simulink library "marine_gnc"  (Simulink 7.4)
settings: Solver=ode45  SolverMode=SingleTasking  StartTime=0.0  StopTime=10.0  RelTol=1e-3
undefined symbols (not defined in the file or in its folder): CN_data, CX_data, CY_data, D, G, K_supply, kt2ms, M, MA, magnitude, marine, Models, MRB, order, pathlength, RAO_Amp, RAO_Dir, RAO_Freq, RAO_Phase, RAO_Vel, RAO_yaw_back, RAO_yaw_quant, RAO_yaw_quantization_flag, rho_a, Semi, sub, T_supply, table, Tanker, vessel, Vessels
libraries: marine_gnc x64, simulink x39, cybersealib x1
(part 4 of 6)

== system marine_gnc/Models/Control Surfaces/Rudder ==
  note: Lift
  note: Drag
  "Alpha_eff " : Inport  OutDataType=sfix(16)  OutScaling=2^0
  Vrel : Inport  Port=2  OutDataType=sfix(16)  OutScaling=2^0
  Constant1 : Constant  Value=CD0  OutDataType=sfix(16)  OutScaling=2^0
  Math Function : Math  Operator=square  OutDataType=sfix(16)  OutScaling=2^0  SaturateOnIntegerOverflow=on
  Mux2 : Mux
  Product1 : Product  Inputs=**  OutDataType=sfix(16)  OutScaling=2^0  SaturateOnIntegerOverflow=on  InputSameDT=on  OutDataTypeStr=Inherit: Same as first input
  Product2 : Product  OutDataType=sfix(16)  OutScaling=2^0  SaturateOnIntegerOverflow=on  InputSameDT=on  OutDataTypeStr=Inherit: Same as first input
  Product4 : Product  OutDataType=sfix(16)  OutScaling=2^0  SaturateOnIntegerOverflow=on  InputSameDT=on  OutDataTypeStr=Inherit: Same as first input
  Saturation : Saturate  UpperLimit=stall  LowerLimit=-stall
  Sum1 : Sum  Inputs=|++  OutDataType=sfix(16)  OutScaling=2^0  SaturateOnIntegerOverflow=on  InputSameDT=on  OutDataTypeStr=Inherit: Same as first input
  "gain " : Gain  Gain=1/(0.9*pi*ar)  ParameterDataType=sfix(16)  ParameterScaling=2^0  OutDataType=sfix(16)  OutScaling=2^0  SaturateOnIntegerOverflow=on  OutDataTypeStr=Inherit: Same as input  ParamDataTypeStr=Inherit: Same as input
  gain 1 : Gain  Gain=dCL  ParameterDataType=sfix(16)  ParameterScaling=2^0  OutDataType=sfix(16)  OutScaling=2^0  SaturateOnIntegerOverflow=on  OutDataTypeStr=Inherit: Same as input  ParamDataTypeStr=Inherit: Same as input
  gain 2 : Gain  Gain=-1  ParameterDataType=sfix(16)  ParameterScaling=2^0  OutDataType=sfix(16)  OutScaling=2^0  SaturateOnIntegerOverflow=on  OutDataTypeStr=Inherit: Same as input  ParamDataTypeStr=Inherit: Same as input
  pi/(2*stall)2 : Gain  Gain=0.5*rho*A  ParameterDataType=sfix(16)  ParameterScaling=2^0  OutDataType=sfix(16)  OutScaling=2^0  SaturateOnIntegerOverflow=on  OutDataTypeStr=Inherit: Same as input  ParamDataTypeStr=Inherit: Same as input
  pi/(2*stall)6 : Gain  Gain=-(VCG-0.5*sp)  ParameterDataType=sfix(16)  ParameterScaling=2^0  OutDataType=sfix(16)  OutScaling=2^0  SaturateOnIntegerOverflow=on  OutDataTypeStr=Inherit: Same as input  ParamDataTypeStr=Inherit: Same as input
  pi/(2*stall)7 : Gain  Gain=-LCG  ParameterDataType=sfix(16)  ParameterScaling=2^0  OutDataType=sfix(16)  OutScaling=2^0  SaturateOnIntegerOverflow=on  OutDataTypeStr=Inherit: Same as input  ParamDataTypeStr=Inherit: Same as input
  "[XYKN]'" : Outport  OutDataType=sfix(16)  OutScaling=2^0
  wires:
  Product1/1 -> pi/(2*stall)2/1
  Vrel/1 -> Product1/2, Product1/1
  Constant1/1 -> Sum1/2
  "gain "/1 -> Sum1/1
  Math Function/1 -> "gain "/1
  Sum1/1 -> Product4/1
  pi/(2*stall)2/1 -> Product2/2, Product4/2
  Product4/1 -> gain 2/1
  gain 2/1 -> Mux2/1
  Mux2/1 -> "[XYKN]'"/1
  pi/(2*stall)6/1 -> Mux2/3
  Product2/1 -> Mux2/2, pi/(2*stall)6/1, pi/(2*stall)7/1
  pi/(2*stall)7/1 -> Mux2/4
  gain 1/1 -> Product2/1, Math Function/1
  Saturation/1 -> gain 1/1
  "Alpha_eff "/1 -> Saturation/1

== system marine_gnc/Models/Control Surfaces/Rudder  forces 4-DOF ==
  Lift : Inport  OutDataType=sfix(16)  OutScaling=2^0
  Drag : Inport  Port=2  OutDataType=sfix(16)  OutScaling=2^0
  Constant : Constant  Value=LCG  OutDataType=sfix(16)  OutScaling=2^0
  Constant2 : Constant  Value=rr  OutDataType=sfix(16)  OutScaling=2^0
  Gain : Gain  Gain=-1  ParameterDataType=sfix(16)  ParameterScaling=2^0  OutDataType=sfix(16)  OutScaling=2^0  SaturateOnIntegerOverflow=on  OutDataTypeStr=Inherit: Same as input  ParamDataTypeStr=Inherit: Same as input
  Gain1 : Gain  Gain=-1  ParameterDataType=sfix(16)  ParameterScaling=2^0  OutDataType=sfix(16)  OutScaling=2^0  SaturateOnIntegerOverflow=on  OutDataTypeStr=Inherit: Same as input  ParamDataTypeStr=Inherit: Same as input
  Product1 : Product  OutDataType=sfix(16)  OutScaling=2^0  SaturateOnIntegerOverflow=on  InputSameDT=on  OutDataTypeStr=Inherit: Same as first input
  Product2 : Product  OutDataType=sfix(16)  OutScaling=2^0  SaturateOnIntegerOverflow=on  InputSameDT=on  OutDataTypeStr=Inherit: Same as first input
  X : Outport  OutDataType=sfix(16)  OutScaling=2^0
  Y : Outport  Port=2  OutDataType=sfix(16)  OutScaling=2^0
  K : Outport  Port=3  OutDataType=sfix(16)  OutScaling=2^0
  N : Outport  Port=4  OutDataType=sfix(16)  OutScaling=2^0
  wires:
  Gain/1 -> X/1
  Drag/1 -> Gain/1
  Gain1/1 -> Product2/1, Product1/1
  Product2/1 -> K/1
  Constant2/1 -> Product2/2
  Lift/1 -> Y/1, Gain1/1
  Constant/1 -> Product1/2
  Product1/1 -> N/1

== system marine_gnc/Models/Control Surfaces/Stabilizer Fins forces 4-DOF ==
  Nf : Inport  OutDataType=sfix(16)  OutScaling=2^0
  Tf : Inport  Port=2  OutDataType=sfix(16)  OutScaling=2^0
  Constant : Constant  Value=FCG  OutDataType=sfix(16)  OutScaling=2^0
  Constant1 : Constant  Value=sinB  OutDataType=sfix(16)  OutScaling=2^0
  Constant2 : Constant  Value=rf  OutDataType=sfix(16)  OutScaling=2^0
  Gain : Gain  Gain=-1  ParameterDataType=sfix(16)  ParameterScaling=2^0  OutDataType=sfix(16)  OutScaling=2^0  SaturateOnIntegerOverflow=on  OutDataTypeStr=Inherit: Same as input  ParamDataTypeStr=Inherit: Same as input
  Gain1 : Gain  Gain=-2  ParameterDataType=sfix(16)  ParameterScaling=2^0  OutDataType=sfix(16)  OutScaling=2^0  SaturateOnIntegerOverflow=on  OutDataTypeStr=Inherit: Same as input  ParamDataTypeStr=Inherit: Same as input
  Product : Product  Inputs=3  OutDataType=sfix(16)  OutScaling=2^0  SaturateOnIntegerOverflow=on  InputSameDT=on  OutDataTypeStr=Inherit: Same as first input
  Product1 : Product  OutDataType=sfix(16)  OutScaling=2^0  SaturateOnIntegerOverflow=on  InputSameDT=on  OutDataTypeStr=Inherit: Same as first input
  Product2 : Product  OutDataType=sfix(16)  OutScaling=2^0  SaturateOnIntegerOverflow=on  InputSameDT=on  OutDataTypeStr=Inherit: Same as first input
  X : Outport  OutDataType=sfix(16)  OutScaling=2^0
  Y : Outport  Port=2  OutDataType=sfix(16)  OutScaling=2^0
  K : Outport  Port=3  OutDataType=sfix(16)  OutScaling=2^0
  N : Outport  Port=4  OutDataType=sfix(16)  OutScaling=2^0
  wires:
  Product1/1 -> Y/1
  Product/1 -> N/1
  Constant/1 -> Product/3
  Constant1/1 -> Product/1, Product1/2
  Nf/1 -> Product/2, Gain1/1, Product1/1
  Constant2/1 -> Product2/2
  Product2/1 -> K/1
  Gain1/1 -> Product2/1
  Tf/1 -> Gain/1
  Gain/1 -> X/1

== system marine_gnc/Models/Control Surfaces/Steady State Hydrofoil ==
  Ang : Inport  OutDataType=sfix(16)  OutScaling=2^0
  "Vf " : Inport  Port=2  OutDataType=sfix(16)  OutScaling=2^0
  Constant1 : Constant  Value=CD0  OutDataType=sfix(16)  OutScaling=2^0
  Gain : Gain  Gain=0.5*rho*A  ParameterDataType=sfix(16)  ParameterScaling=2^0  OutDataType=sfix(16)  OutScaling=2^0  SaturateOnIntegerOverflow=on  OutDataTypeStr=Inherit: Same as input  ParamDataTypeStr=Inherit: Same as input
  Lookup Table CL(Ang) : Lookup  InputValues=AE  Table=CLAE  LookUpMeth=Interpolation-Use End Values  OutDataType=sfix(16)  OutScaling=2^0
  Math Function : Math  Operator=square  OutDataType=sfix(16)  OutScaling=2^0  SaturateOnIntegerOverflow=on
  Product{1,3,5..7} (5 alike) : Product  Inputs=**  OutDataType=sfix(16)  OutScaling=2^0  SaturateOnIntegerOverflow=on  InputSameDT=on  OutDataTypeStr=Inherit: Same as first input
  Product2 : Product  OutDataType=sfix(16)  OutScaling=2^0  SaturateOnIntegerOverflow=on  InputSameDT=on  OutDataTypeStr=Inherit: Same as first input
  Product4 : Product  OutDataType=sfix(16)  OutScaling=2^0  SaturateOnIntegerOverflow=on  InputSameDT=on  OutDataTypeStr=Inherit: Same as first input
  Saturation : Saturate  UpperLimit=AM  LowerLimit=-AM
  Sum1 : Sum  Inputs=|++  OutDataType=sfix(16)  OutScaling=2^0  SaturateOnIntegerOverflow=on  InputSameDT=on  OutDataTypeStr=Inherit: Same as first input
  Sum2 : Sum  Inputs=|++  OutDataType=sfix(16)  OutScaling=2^0  SaturateOnIntegerOverflow=on  InputSameDT=on  OutDataTypeStr=Inherit: Same as first input
  Sum3 : Sum  Inputs=|-+  OutDataType=sfix(16)  OutScaling=2^0  SaturateOnIntegerOverflow=on  InputSameDT=on  OutDataTypeStr=Inherit: Same as first input
  Trigonometric Function : Trigonometry  Operator=cos
  Trigonometric Function1 : Trigonometry
  "gain " : Gain  Gain=1/(0.9*pi*ar)  ParameterDataType=sfix(16)  ParameterScaling=2^0  OutDataType=sfix(16)  OutScaling=2^0  SaturateOnIntegerOverflow=on  OutDataTypeStr=Inherit: Same as input  ParamDataTypeStr=Inherit: Same as input
  Lift : Outport  OutDataType=sfix(16)  OutScaling=2^0
  Drag : Outport  Port=2  OutDataType=sfix(16)  OutScaling=2^0
  N : Outport  Port=3  OutDataType=sfix(16)  OutScaling=2^0
  T : Outport  Port=4  OutDataType=sfix(16)  OutScaling=2^0
  wires:
  Lookup Table CL(Ang)/1 -> Math Function/1, Product2/1
  Product4/1 -> Drag/1, Product5/1, Product6/1
  Gain/1 -> Product2/2, Product4/2
  Sum1/1 -> Product4/1
  Math Function/1 -> "gain "/1
  "gain "/1 -> Sum1/1
  Constant1/1 -> Sum1/2
  "Vf "/1 -> Product1/1, Product1/2
  Product1/1 -> Gain/1
  Product2/1 -> Lift/1, Product3/1, Product7/1
  Product3/1 -> Sum2/1
  Product5/1 -> Sum2/2
  Trigonometric Function/1 -> Product3/2, Product6/2
  Trigonometric Function1/1 -> Product5/2, Product7/2
  Sum2/1 -> N/1
  Product6/1 -> Sum3/1
  Product7/1 -> Sum3/2
  Sum3/1 -> T/1
  Saturation/1 -> Lookup Table CL(Ang)/1
  Ang/1 -> Saturation/1, Trigonometric Function1/1, Trigonometric Function/1

== system marine_gnc/Models/Environmental Loads/Force RAO ==
  eta : Inport  OutDataType=sfix(16)  OutScaling=2^0
  U : Inport  Port=2  OutDataType=sfix(16)  OutScaling=2^0
  Waves : Inport  Port=3  OutDataType=sfix(16)  OutScaling=2^0
  Abs : Abs
  Backlash : Backlash  BacklashWidth=RAO_speed_back
  Bus Selector : BusSelector  OutputSignals=Psi,Wavenum,Omega,Phase,Zeta_a
  Clock : Clock
      settings: Decimation=10
  Omega range error : marine_gnc/Utilities/Simulation tools/Signal range error  Values=RAO_Freq  message=Wave frequency outside range of RAO table
  Output smoothing flag : Constant  Value=RAO_smoothing_flag  OutDataType=sfix(16)  OutScaling=2^0
  Position phase : marine_gnc/Models/Environmental Loads/Utilities/Position phase
  Product1 : Product  Inputs=**  OutDataType=sfix(16)  OutScaling=2^0  SaturateOnIntegerOverflow=on  OutDataTypeStr=Inherit: Same as first input
  Psi_r range error : marine_gnc/Utilities/Simulation tools/Signal range error  Values=RAO_Dir  message=Relative wave direction outside range of RAO table
  Signal smoothing : marine_gnc/Models/Environmental Loads/Utilities/Signal smoothing
  Speed lookup table : Lookup  InputValues=RAO_Vel  Table=RAO_Vel  LookUpMeth=Use Input Nearest  OutDataType=sfix(16)  OutScaling=2^0
  Speed quantizer flag : Constant  Value=RAO_speed_backlash_flag  OutDataType=sfix(16)  OutScaling=2^0
  Sum : Sum  Inputs=-++  OutDataType=sfix(16)  OutScaling=2^0  SaturateOnIntegerOverflow=on
  Switch1 : Switch  Threshold=0.5
  Switch2 : Switch  Threshold=0.5
  Wave component loop : Subsystem  TreatAsAtomicUnit=on
  Width : Width  DataType=int32
  Yaw quantizer : marine_gnc/Models/Environmental Loads/Utilities/Yaw quantizer  quant_flag=RAO_yaw_quantization_flag  quant=RAO_yaw_quant  back=RAO_yaw_back
  "[-inf inf] to [-pi pi]" : marine_gnc/Utilities/Math Operations/[-inf inf] to [-pi pi]
  yaw angle : Selector  InputPortWidth=6  IndexOptions=Index vector (dialog)  Indices=6  OutputSizes=1
  tau WF : Outport  OutDataType=sfix(16)  OutScaling=2^0
  wires:
  Wave component loop/2(Tau rate) -> Signal smoothing/2
  Signal smoothing/1 -> Switch2/1
  Wave component loop/1(Tau WF) -> Signal smoothing/1, Switch2/3
  Switch2/1 -> tau WF/1
  Output smoothing flag/1 -> Switch2/2
  Abs/1 -> Psi_r range error/1
  "[-inf inf] to [-pi pi]"/1 -> Abs/1, Wave component loop/2(Psi_r)
  eta/1 -> yaw angle/1, Position phase/3
  Bus Selector/2 -> Position phase/2  "<Wavenum>"
  Bus Selector/4 -> Sum/3  "<Phase>"
  Waves/1 -> Bus Selector/1
  Product1/1 -> Sum/2
  Bus Selector/1 -> Position phase/1, Yaw quantizer/2  "<Psi>"
  Clock/1 -> Product1/2
  Bus Selector/3 -> Wave component loop/3(Omega), Omega range error/1, Width/1, Product1/1  "<Omega>"
  Sum/1 -> Wave component loop/4(Phase_tot)  "Phase_tot"
  Bus Selector/5 -> Wave component loop/5(Zeta_a)  "<Zeta_a>"
  Width/1 -> Wave component loop/1(number of  iterations)
  U/1 -> Backlash/1, Switch1/3
  Position phase/1 -> Sum/1
  Yaw quantizer/1 -> "[-inf inf] to [-pi pi]"/1
  yaw angle/1 -> Yaw quantizer/1
  Speed quantizer flag/1 -> Switch1/2
  Backlash/1 -> Switch1/1
  Switch1/1 -> Speed lookup table/1
  Speed lookup table/1 -> Wave component loop/6(U)

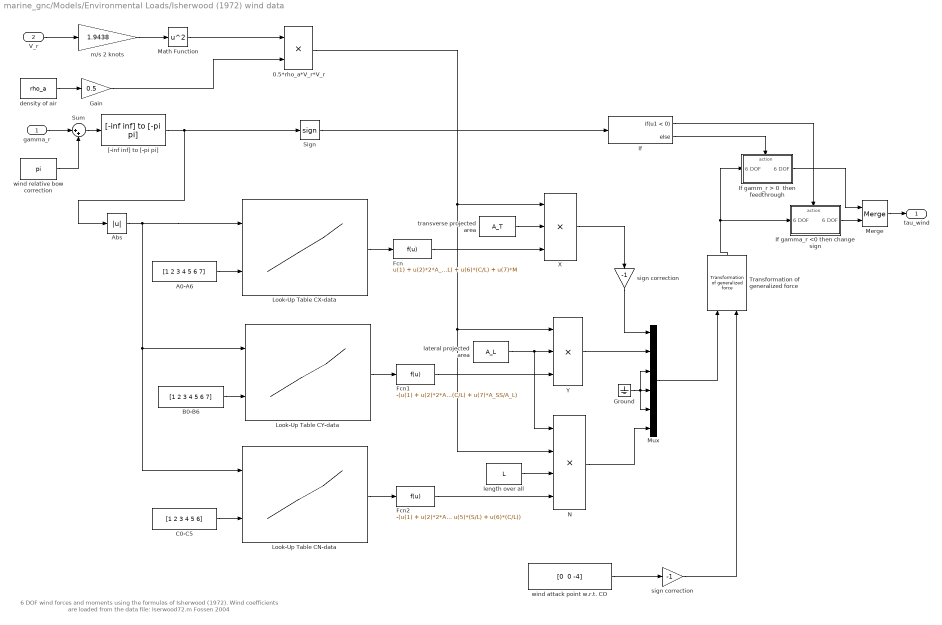
== system marine_gnc/Models/Environmental Loads/Isherwood (1972) wind data ==
  note: 6 DOF wind forces and moments using the formulas of Isherwood (1972).
      | Wind coefficients are loaded from the data file: Iserwood72.m
      |
      | Fossen 2004
  gamma_r : Inport  OutDataType=sfix(16)  OutScaling=2^0
  V_r : Inport  Port=2  OutDataType=sfix(16)  OutScaling=2^0
  0.5*rho_a*V_r*V_r : Product  OutDataType=sfix(16)  OutScaling=2^0  SaturateOnIntegerOverflow=on  OutDataTypeStr=Inherit: Same as first input
  A0-A6 : Constant  Value=[1 2 3 4 5 6 7]  OutDataType=sfix(16)  OutScaling=2^0
  Abs : Abs  SaturateOnIntegerOverflow=on
  B0-B6 : Constant  Value=[1 2 3 4 5 6 7]  OutDataType=sfix(16)  OutScaling=2^0
  C0-C5 : Constant  Value=[1 2 3 4 5 6]  OutDataType=sfix(16)  OutScaling=2^0
  Fcn : Fcn  Expr=u(1) + u(2)*2*A_L/L^2 + u(3)*2*A_T/B^2 + u(4)*(L/B) + u(5)*(S/L) + u(6)*(C/L) + u(7)*M
  Fcn1 : Fcn  Expr=-(u(1) + u(2)*2*A_L/L^2 + u(3)*2*A_T/B^2 + u(4)*(L/B) + u(5)*(S/L) + u(6)*(C/L) + u(7)*A_SS/A_L)
  Fcn2 : Fcn  Expr=-(u(1) + u(2)*2*A_L/L^2 + u(3)*2*A_T/B^2 + u(4)*(L/B) + u(5)*(S/L) + u(6)*(C/L))
  Gain : Gain  Gain=0.5  ParameterDataType=sfix(16)  ParameterScaling=2^0  OutDataType=sfix(16)  OutScaling=2^0  SaturateOnIntegerOverflow=on  OutDataTypeStr=Inherit: Same as input  ParamDataTypeStr=Inherit: Same as input
  Ground : Ground
  If : If  IfExpression=u1 < 0
  If gamm_r > 0  then feedthrough : Subsystem  TreatAsAtomicUnit=on
  If gamma_r <0 then change sign : Subsystem  TreatAsAtomicUnit=on
  Look-Up Table CN-data : Lookup2D  RowIndex=gamma_r_iserwood  ColumnIndex=[1:6]  Table=CN_data  OutDataTypeMode=double  OutDataType=sfix(16)  OutScaling=2^0  OutDataTypeStr=double  SaturateOnIntegerOverflow=on
  Look-Up Table CX-data : Lookup2D  RowIndex=gamma_r_iserwood  ColumnIndex=[1:7]  Table=CX_data  OutDataTypeMode=double  OutDataType=sfix(16)  OutScaling=2^0  OutDataTypeStr=double  SaturateOnIntegerOverflow=on
  Look-Up Table CY-data : Lookup2D  RowIndex=gamma_r_iserwood  ColumnIndex=[1:7]  Table=CY_data  OutDataTypeMode=double  OutDataType=sfix(16)  OutScaling=2^0  OutDataTypeStr=double  SaturateOnIntegerOverflow=on
  Math Function : Math  Operator=square  OutDataType=sfix(16)  OutScaling=2^0  SaturateOnIntegerOverflow=on
  Merge : Merge
  Mux : Mux  Inputs=6
  N : Product  Inputs=4  OutDataType=sfix(16)  OutScaling=2^0  SaturateOnIntegerOverflow=on  OutDataTypeStr=Inherit: Same as first input
  Sign : Signum
  Sum : Sum  Inputs=|++  OutDataType=sfix(16)  OutScaling=2^0  SaturateOnIntegerOverflow=on
  Transformation of generalized force : marine_gnc/Models/ Kinematics/Transformation of generalized force
  X : Product  Inputs=3  OutDataType=sfix(16)  OutScaling=2^0  SaturateOnIntegerOverflow=on  OutDataTypeStr=Inherit: Same as first input
  Y : Product  Inputs=3  OutDataType=sfix(16)  OutScaling=2^0  SaturateOnIntegerOverflow=on  OutDataTypeStr=Inherit: Same as first input
  "[-inf inf] to [-pi pi]" : marine_gnc/Utilities/Math Operations/[-inf inf] to [-pi pi]
  density of air : Constant  Value=rho_a  OutDataType=sfix(16)  OutScaling=2^0
  lateral projected area : Constant  Value=A_L  OutDataType=sfix(16)  OutScaling=2^0
  length over all : Constant  Value=L  OutDataType=sfix(16)  OutScaling=2^0
  m/s 2 knots : Gain  Gain=1.9438  ParameterDataType=sfix(16)  ParameterScaling=2^0  OutDataType=sfix(16)  OutScaling=2^0  SaturateOnIntegerOverflow=on  OutDataTypeStr=Inherit: Same as input  ParamDataTypeStr=Inherit: Same as input
  sign correction : Gain  Gain=-1  ParameterDataType=sfix(16)  ParameterScaling=2^0  OutDataType=sfix(16)  OutScaling=2^0  SaturateOnIntegerOverflow=on  OutDataTypeStr=Inherit: Same as input  ParamDataTypeStr=Inherit: Same as input
  "sign correction " : Gain  Gain=-1  ParameterDataType=sfix(16)  ParameterScaling=2^0  OutDataType=sfix(16)  OutScaling=2^0  SaturateOnIntegerOverflow=on  OutDataTypeStr=Inherit: Same as input  ParamDataTypeStr=Inherit: Same as input
  transverse projected area : Constant  Value=A_T  OutDataType=sfix(16)  OutScaling=2^0
  wind attack point w.r.t. CO : Constant  Value="[0  0 -4]"  OutDataType=sfix(16)  OutScaling=2^0
  wind relative bow correction : Constant  Value=pi  OutDataType=sfix(16)  OutScaling=2^0
  tau_wind : Outport  OutDataType=sfix(16)  OutScaling=2^0
  wires:
  sign correction/1 -> Mux/1
  "[-inf inf] to [-pi pi]"/1 -> Sign/1, Abs/1
  Sum/1 -> "[-inf inf] to [-pi pi]"/1
  wind relative bow correction/1 -> Sum/2
  Ground/1 -> Mux/5, Mux/4, Mux/3
  Mux/1 -> Transformation of generalized force/1
  Merge/1 -> tau_wind/1
  "sign correction "/1 -> Transformation of generalized force/2
  wind attack point w.r.t. CO/1 -> "sign correction "/1
  Sign/1 -> If/1
  If gamm_r > 0  then feedthrough/1("6 DOF  ") -> Merge/1
  If gamma_r <0 then change sign/1("6 DOF  ") -> Merge/2
  If/1 -> If gamma_r <0 then change sign/Action
  If/2 -> If gamm_r > 0  then feedthrough/Action
  Transformation of generalized force/1 -> If gamm_r > 0  then feedthrough/1(6 DOF), If gamma_r <0 then change sign/1(6 DOF)
  Abs/1 -> Look-Up Table CN-data/1, Look-Up Table CY-data/1, Look-Up Table CX-data/1
  m/s 2 knots/1 -> Math Function/1
  length over all/1 -> N/3
  N/1 -> Mux/6
  Y/1 -> Mux/2
  lateral projected area/1 -> N/1, Y/2
  X/1 -> sign correction/1
  transverse projected area/1 -> X/2
  0.5*rho_a*V_r*V_r/1 -> N/2, Y/1, X/1
  Gain/1 -> 0.5*rho_a*V_r*V_r/2
  Math Function/1 -> 0.5*rho_a*V_r*V_r/1
  V_r/1 -> m/s 2 knots/1
  density of air/1 -> Gain/1
  Fcn2/1 -> N/4
  Fcn1/1 -> Y/3
  Fcn/1 -> X/3
  gamma_r/1 -> Sum/1
  Look-Up Table CN-data/1 -> Fcn2/1
  Look-Up Table CY-data/1 -> Fcn1/1
  C0-C5/1 -> Look-Up Table CN-data/2
  B0-B6/1 -> Look-Up Table CY-data/2
  Look-Up Table CX-data/1 -> Fcn/1
  A0-A6/1 -> Look-Up Table CX-data/2

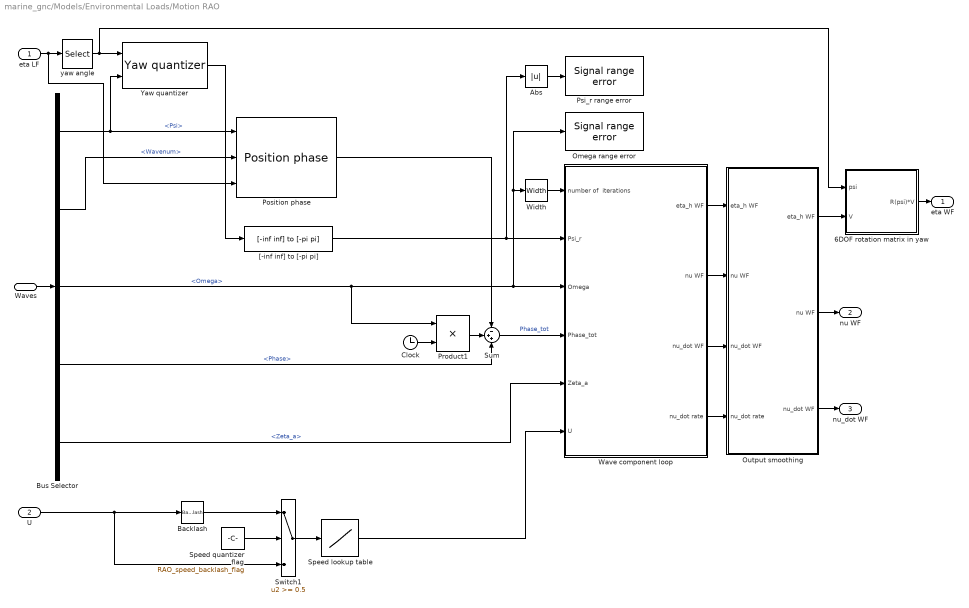
== system marine_gnc/Models/Environmental Loads/Motion RAO ==
  eta LF : Inport  OutDataType=sfix(16)  OutScaling=2^0
  U : Inport  Port=2  OutDataType=sfix(16)  OutScaling=2^0
  Waves : Inport  Port=3  OutDataType=sfix(16)  OutScaling=2^0
  6DOF rotation matrix in yaw : Subsystem
  Abs : Abs
  Backlash : Backlash  BacklashWidth=RAO_speed_back
  Bus Selector : BusSelector  OutputSignals=Psi,Wavenum,Omega,Phase,Zeta_a
  Clock : Clock
      settings: Decimation=10
  Omega range error : marine_gnc/Utilities/Simulation tools/Signal range error  Values=RAO_Freq  message=Wave frequency outside range of RAO table
  Output smoothing : Subsystem
  Position phase : marine_gnc/Models/Environmental Loads/Utilities/Position phase
  Product1 : Product  Inputs=**  OutDataType=sfix(16)  OutScaling=2^0  SaturateOnIntegerOverflow=on  OutDataTypeStr=Inherit: Same as first input
  Psi_r range error : marine_gnc/Utilities/Simulation tools/Signal range error  Values=RAO_Dir  message=Relative wave direction outside range of RAO table
  Speed lookup table : Lookup  InputValues=RAO_Vel  Table=RAO_Vel  LookUpMeth=Use Input Nearest  OutDataType=sfix(16)  OutScaling=2^0
  Speed quantizer flag : Constant  Value=RAO_speed_backlash_flag  OutDataType=sfix(16)  OutScaling=2^0
  Sum : Sum  Inputs=-++  OutDataType=sfix(16)  OutScaling=2^0  SaturateOnIntegerOverflow=on
  Switch1 : Switch  Threshold=0.5
  Wave component loop : Subsystem  TreatAsAtomicUnit=on
  Width : Width  DataType=int32
  Yaw quantizer : marine_gnc/Models/Environmental Loads/Utilities/Yaw quantizer  quant_flag=RAO_yaw_quantization_flag  quant=RAO_yaw_quant  back=RAO_yaw_back
  "[-inf inf] to [-pi pi]" : marine_gnc/Utilities/Math Operations/[-inf inf] to [-pi pi]
  yaw angle : Selector  InputPortWidth=6  IndexOptions=Index vector (dialog)  Indices=6  OutputSizes=1
  eta WF : Outport  OutDataType=sfix(16)  OutScaling=2^0
  nu WF : Outport  Port=2  OutDataType=sfix(16)  OutScaling=2^0
  nu_dot WF : Outport  Port=3  OutDataType=sfix(16)  OutScaling=2^0
  wires:
  Output smoothing/1("eta_h WF ") -> 6DOF rotation matrix in yaw/2(V)
  Wave component loop/4(nu_dot rate) -> Output smoothing/4(nu_dot rate)
  Wave component loop/1(eta_h WF) -> Output smoothing/1(eta_h WF)
  Output smoothing/3(nu_dot WF) -> nu_dot WF/1
  Output smoothing/2(nu WF) -> nu WF/1
  eta LF/1 -> yaw angle/1, Position phase/3
  Bus Selector/2 -> Position phase/2  "<Wavenum>"
  Bus Selector/4 -> Sum/3  "<Phase>"
  Waves/1 -> Bus Selector/1
  Product1/1 -> Sum/2
  Bus Selector/1 -> Position phase/1, Yaw quantizer/2  "<Psi>"
  Clock/1 -> Product1/2
  yaw angle/1 -> 6DOF rotation matrix in yaw/1(psi), Yaw quantizer/1
  Bus Selector/3 -> Wave component loop/3(Omega), Width/1, Omega range error/1, Product1/1  "<Omega>"
  6DOF rotation matrix in yaw/1(R(psi)*V) -> eta WF/1
  Sum/1 -> Wave component loop/4(Phase_tot)  "Phase_tot"
  Bus Selector/5 -> Wave component loop/5(Zeta_a)  "<Zeta_a>"
  Width/1 -> Wave component loop/1(number of  iterations)
  U/1 -> Backlash/1, Switch1/3
  Wave component loop/2(nu WF) -> Output smoothing/2("nu WF ")
  Wave component loop/3(nu_dot WF) -> Output smoothing/3("nu_dot WF ")
  Abs/1 -> Psi_r range error/1
  Yaw quantizer/1 -> "[-inf inf] to [-pi pi]"/1
  "[-inf inf] to [-pi pi]"/1 -> Wave component loop/2(Psi_r), Abs/1
  Speed quantizer flag/1 -> Switch1/2
  Backlash/1 -> Switch1/1
  Switch1/1 -> Speed lookup table/1
  Speed lookup table/1 -> Wave component loop/6(U)
  Position phase/1 -> Sum/1

== system marine_gnc/Models/Environmental Loads/Utilities ==
  Position phase : Subsystem
      mask Type: Position Phase
      mask Description: Calculate the phase delay due to the vessel LF position.
  RAO tables : Subsystem  mask(RAO table lookup){RAO_Freq=RAO_Freq, RAO_Dir=RAO_Dir, RAO_Vel=RAO_Vel, RAO_Amp=RAO_Amp, RAO_Phase=RAO_Phase}
      mask prompts: RAO_Freq "Vector of frequencies (rad/s)"; RAO_Dir "Vector of directions (rad)"; RAO_Vel "Vector of velocities (m/s)"; RAO_Amp "6DOF Cell array with tables of Amplitudes"; RAO_Phase "6DOF Cell array with tables of Phases (rad)"
      mask help:
      | Perform 3D table lookup in 6DOF RAO amplitudes and phases, using the relative wave heading psi_r, wave frequency omega and vessel velocity vel as inputs. See documentation of the Motion RAO block or Force RAO block for details. A warning is issued if the input is outside the range spanned by the RAOs.
      |
      | Copyright (C) NTNU 2005
      |
      | Author: Oyvind N. Smogeli, 2005-05-03
  Signal smoothing : Subsystem
      mask Type: Signal smoothing
      mask Description:
      | Rate limit the input signal according to the recorded maximum signal rate.
      | 
      | For example, in order to remove switching transients from a velocity signal, input the acceleration signal as signal rate.
  Yaw quantizer : Subsystem  mask(Yaw quantizer){quant_flag=RAO_yaw_quantization_flag, quant=RAO_yaw_quant, back=RAO_yaw_back}
      mask prompts: quant_flag "Quantizer flag {0,1}"; quant "Quantizer interval [rad]"; back "Backlash width [rad]"
      mask help: Apply quantization and backlash to the yaw angle if desired, and calculate the wave direction relative to the vessel. If the quantizer flag is set to zero, the two outputs are equal.

== system marine_gnc/Models/Propulsion/Actuator Configuration ==
  2 main propellers and 3 tunnel  thrusters : Subsystem
      mask Display: disp('tau = T*K(n)*u')
  "2 main propellers, 1 azimuth and 2 tunnel thrusters" : Subsystem
      mask Display:
      | disp('tau =            \n\n')
      | disp('    T(alpha)*K(n)*u')
  4 azimuth thrusters : Subsystem
      mask Display:
      | disp('tau =            \n\n')
      | disp('    T(alpha)*K(n)*u')
  Column vector t : Subsystem
  Thruster configuration matrix : Subsystem

== system marine_gnc/Models/Propulsion/Open-water propeller characteristics ==
  n : Inport  OutDataType=sfix(16)  OutScaling=2^0
  Va : Inport  Port=2  OutDataType=sfix(16)  OutScaling=2^0
  Dot Product1 : simulink/Math Operations/Dot Product  InputSameDT=on  OutDataType=sfix(16)  OutScaling=2^-10  DoSatur=off
  Dot Product2 : simulink/Math Operations/Dot Product  InputSameDT=on  OutDataType=sfix(16)  OutScaling=2^-10  DoSatur=off
  Kq poly : Constant  Value=Par_Thruster_Kqp  OutDataType=sfix(16)  OutScaling=2^0
  Kt poly : Constant  Value=Par_Thruster_Ktp  OutDataType=sfix(16)  OutScaling=2^0
  Math Function3 : Math  Operator=magnitude^2  OutDataType=sfix(16)  OutScaling=2^0  SaturateOnIntegerOverflow=on
  Math Function4 : Math  Operator=magnitude^2  OutDataType=sfix(16)  OutScaling=2^0  SaturateOnIntegerOverflow=on
  Mux1 : Mux  Inputs=3
  Product{2..3,6,9..10} (5 alike) : Product  OutDataType=sfix(16)  OutScaling=2^0  SaturateOnIntegerOverflow=on  OutDataTypeStr=Inherit: Same as first input
  Sign : Signum
  Switch : Switch  SaturateOnIntegerOverflow=on
  Zero limit : Saturate  UpperLimit=inf  LowerLimit=0
  Zero limit1 : Saturate  UpperLimit=inf  LowerLimit=0
  Zero limit2 : Saturate  UpperLimit=inf  LowerLimit=0
  reverse reduction : Gain  Gain=Par_Thruster_reverse_reduction  ParameterDataType=sfix(16)  ParameterScaling=2^0  OutDataType=sfix(16)  OutScaling=2^0  SaturateOnIntegerOverflow=on  OutDataTypeStr=Inherit: Same as input  ParamDataTypeStr=Inherit: Same as input
  rhow[D^2 D^3 D^4] : Constant  Value=Glob_rhow*[Par_Thruster_D^2 Par_Thruster_D^3 Par_Thruster_D^4]  OutDataType=sfix(16)  OutScaling=2^0
  "rhow[D^3 D^4 D^5] " : Constant  Value=Glob_rhow*[Par_Thruster_D^3 Par_Thruster_D^4 Par_Thruster_D^5]  OutDataType=sfix(16)  OutScaling=2^0
  T_a : Outport  OutDataType=sfix(16)  OutScaling=2^0
  Q_a : Outport  Port=2  OutDataType=sfix(16)  OutScaling=2^0
  wires:
  Product10/1 -> Mux1/2
  Math Function4/1 -> Mux1/3
  Math Function3/1 -> Mux1/1
  n/1 -> Sign/1, Product10/2, Math Function4/1
  Product9/1 -> Dot Product2/2
  "rhow[D^3 D^4 D^5] "/1 -> Product9/2
  Kq poly/1 -> Product9/1
  Product6/1 -> Dot Product1/1
  rhow[D^2 D^3 D^4]/1 -> Product6/2
  Kt poly/1 -> Product6/1
  Sign/1 -> Product3/2, Switch/2, Product2/2
  Va/1 -> Zero limit2/1
  Zero limit1/1 -> Product3/1
  Zero limit/1 -> Product2/1
  Dot Product2/1 -> Zero limit1/1
  Dot Product1/1 -> Zero limit/1
  Product3/1 -> Q_a/1
  Product2/1 -> Switch/1, reverse reduction/1
  Switch/1 -> T_a/1
  reverse reduction/1 -> Switch/3
  Mux1/1 -> Dot Product1/2
  Zero limit2/1 -> Math Function3/1, Product10/1

== system marine_gnc/Models/Propulsion/Propeller shaft dynamics ==
  RPM_c : Inport  OutDataType=sfix(16)  OutScaling=2^0
  Gain : Gain  Gain=1/tc  ParameterDataType=sfix(16)  ParameterScaling=2^0  OutDataType=sfix(16)  OutScaling=2^0  SaturateOnIntegerOverflow=on  OutDataTypeStr=Inherit: Same as input  ParamDataTypeStr=Inherit: Same as input
  Integrator1 : Integrator
  Saturation : Saturate  UpperLimit=rpm_rate  LowerLimit=-rpm_rate
  Saturation1 : Saturate  UpperLimit=rpm_max  LowerLimit=-rpm_max
  Sum1 : Sum  Inputs=|+-  OutDataType=sfix(16)  OutScaling=2^0  SaturateOnIntegerOverflow=on  InputSameDT=on  OutDataTypeStr=Inherit: Same as first input
  RPM : Outport  OutDataType=sfix(16)  OutScaling=2^0
  wires:
  RPM_c/1 -> Saturation1/1
  Saturation/1 -> Integrator1/1
  Saturation1/1 -> Sum1/1
  Integrator1/1 -> Sum1/2, RPM/1
  Sum1/1 -> Gain/1
  Gain/1 -> Saturation/1

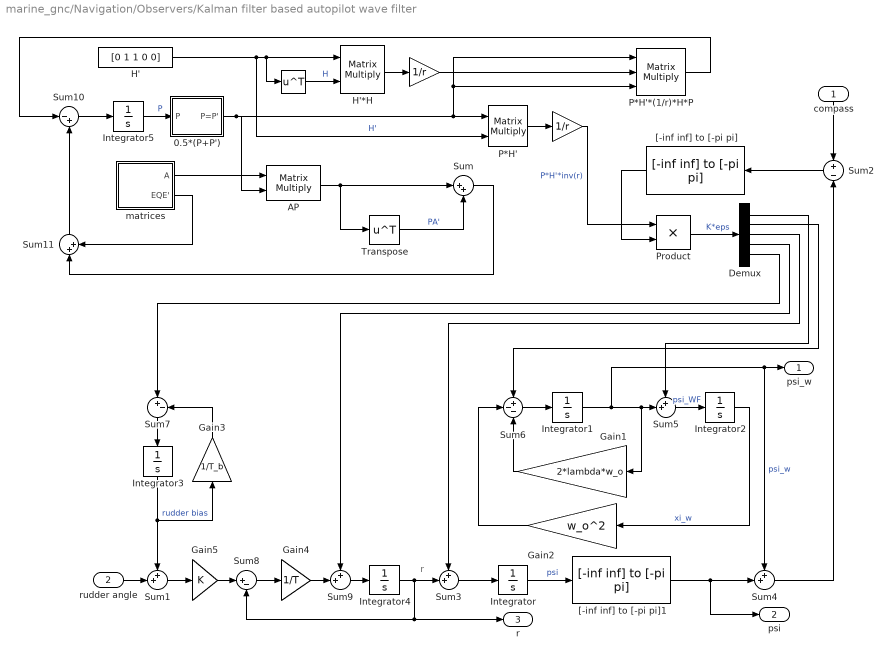
== system marine_gnc/Navigation/Observers/Kalman filter based autopilot wave filter ==
  note: r
  compass : Inport  OutDataType=sfix(16)  OutScaling=2^0
  rudder angle : Inport  Port=2  OutDataType=sfix(16)  OutScaling=2^0
  "  " : Math  Operator=transpose  OutDataType=sfix(16)  OutScaling=2^0  SaturateOnIntegerOverflow=on
  "    " : Gain  Gain=1/r  ParameterDataType=sfix(16)  ParameterScaling=2^0  OutDataType=sfix(16)  OutScaling=2^0  SaturateOnIntegerOverflow=on  OutDataTypeStr=Inherit: Same as input  ParamDataTypeStr=Inherit: Same as input
  "     " : Gain  Gain=1/r  ParameterDataType=sfix(16)  ParameterScaling=2^0  OutDataType=sfix(16)  OutScaling=2^0  SaturateOnIntegerOverflow=on  OutDataTypeStr=Inherit: Same as input  ParamDataTypeStr=Inherit: Same as input
  0.5*(P+P') : Subsystem
  AP : Product  Multiplication=Matrix(*)  OutDataType=sfix(16)  OutScaling=2^0  SaturateOnIntegerOverflow=on  OutDataTypeStr=Inherit: Same as first input
  Demux : Demux  Outputs=5
  Gain1 : Gain  Gain=2*lambda*w_o  ParameterDataType=sfix(16)  ParameterScaling=2^0  OutDataType=sfix(16)  OutScaling=2^0  SaturateOnIntegerOverflow=on  OutDataTypeStr=Inherit: Same as input  ParamDataTypeStr=Inherit: Same as input
  Gain2 : Gain  Gain=w_o^2  ParameterDataType=sfix(16)  ParameterScaling=2^0  OutDataType=sfix(16)  OutScaling=2^0  SaturateOnIntegerOverflow=on  OutDataTypeStr=Inherit: Same as input  ParamDataTypeStr=Inherit: Same as input
  Gain3 : Gain  Gain=1/T_b  ParameterDataType=sfix(16)  ParameterScaling=2^0  OutDataType=sfix(16)  OutScaling=2^0  SaturateOnIntegerOverflow=on  OutDataTypeStr=Inherit: Same as input  ParamDataTypeStr=Inherit: Same as input
  Gain4 : Gain  Gain=1/T  ParameterDataType=sfix(16)  ParameterScaling=2^0  OutDataType=sfix(16)  OutScaling=2^0  SaturateOnIntegerOverflow=on  OutDataTypeStr=Inherit: Same as input  ParamDataTypeStr=Inherit: Same as input
  Gain5 : Gain  Gain=K  ParameterDataType=sfix(16)  ParameterScaling=2^0  OutDataType=sfix(16)  OutScaling=2^0  SaturateOnIntegerOverflow=on  OutDataTypeStr=Inherit: Same as input  ParamDataTypeStr=Inherit: Same as input
  H' : Constant  Value=[0 1 1 0 0]  OutDataType=sfix(16)  OutScaling=2^0
  H'*H : Product  Multiplication=Matrix(*)  OutDataType=sfix(16)  OutScaling=2^0  SaturateOnIntegerOverflow=on  OutDataTypeStr=Inherit: Same as first input
  Integrator{,1..4} (5 alike) : Integrator
  Integrator5 : Integrator  InitialCondition=P0
  P*H' : Product  Inputs=**  Multiplication=Matrix(*)  OutDataType=sfix(16)  OutScaling=2^0  SaturateOnIntegerOverflow=on  OutDataTypeStr=Inherit: Same as first input
  P*H'*(1/r)*H*P : Product  Inputs=***  Multiplication=Matrix(*)  OutDataType=sfix(16)  OutScaling=2^0  SaturateOnIntegerOverflow=on  OutDataTypeStr=Inherit: Same as first input
  Product : Product  OutDataType=sfix(16)  OutScaling=2^0  SaturateOnIntegerOverflow=on  OutDataTypeStr=Inherit: Same as first input
  Sum : Sum  Inputs=|++  OutDataType=sfix(16)  OutScaling=2^0  SaturateOnIntegerOverflow=on
  Sum{1,3..5,9} (5 alike) : Sum  Inputs=++|  OutDataType=sfix(16)  OutScaling=2^0  SaturateOnIntegerOverflow=on  InputSameDT=on  OutDataTypeStr=Inherit: Same as first input
  Sum10 : Sum  Inputs=|-+  OutDataType=sfix(16)  OutScaling=2^0  SaturateOnIntegerOverflow=on
  Sum11 : Sum  Inputs=|++  OutDataType=sfix(16)  OutScaling=2^0  SaturateOnIntegerOverflow=on
  Sum2 : Sum  Inputs=+|-  OutDataType=sfix(16)  OutScaling=2^0  SaturateOnIntegerOverflow=on  InputSameDT=on  OutDataTypeStr=Inherit: Same as first input
  Sum6 : Sum  Inputs=+--  OutDataType=sfix(16)  OutScaling=2^0  SaturateOnIntegerOverflow=on  InputSameDT=on  OutDataTypeStr=Inherit: Same as first input
  Sum7 : Sum  Inputs=|+-  OutDataType=sfix(16)  OutScaling=2^0  SaturateOnIntegerOverflow=on  InputSameDT=on  OutDataTypeStr=Inherit: Same as first input
  Sum8 : Sum  Inputs=|+-  OutDataType=sfix(16)  OutScaling=2^0  SaturateOnIntegerOverflow=on  InputSameDT=on  OutDataTypeStr=Inherit: Same as first input
  Transpose : Math  Operator=transpose  OutDataType=sfix(16)  OutScaling=2^0  SaturateOnIntegerOverflow=on
  "[-inf inf] to [-pi pi]" : marine_gnc/Utilities/Math Operations/[-inf inf] to [-pi pi]
  "[-inf inf] to [-pi pi]1" : marine_gnc/Utilities/Math Operations/[-inf inf] to [-pi pi]
  matrices : Subsystem
  psi_w : Outport  OutDataType=sfix(16)  OutScaling=2^0
  psi : Outport  Port=2  OutDataType=sfix(16)  OutScaling=2^0
  r : Outport  Port=3  OutDataType=sfix(16)  OutScaling=2^0
  wires:
  0.5*(P+P')/1(P=P') -> P*H'*(1/r)*H*P/1, P*H'*(1/r)*H*P/3, P*H'/1, AP/2
  Integrator5/1 -> 0.5*(P+P')/1(P)  "P"
  P*H'*(1/r)*H*P/1 -> Sum10/1
  Demux/4 -> Sum9/1
  Demux/3 -> Sum3/1
  Demux/2 -> Sum6/1
  Demux/1 -> Sum5/1
  Product/1 -> Demux/1  "K*eps"
  "[-inf inf] to [-pi pi]"/1 -> Product/2
  Sum/1 -> Sum11/1
  matrices/2(EQE') -> Sum11/2
  "     "/1 -> Product/1  "P*H'*inv(r)"
  Sum11/1 -> Sum10/2
  Transpose/1 -> Sum/2  "PA'"
  Sum10/1 -> Integrator5/1
  AP/1 -> Transpose/1, Sum/1
  Sum9/1 -> Integrator4/1
  Gain4/1 -> Sum9/2
  Gain5/1 -> Sum8/1
  Gain3/1 -> Sum7/2
  Integrator3/1 -> Gain3/1, Sum1/1  "rudder bias"
  Sum7/1 -> Integrator3/1
  Demux/5 -> Sum7/1
  Integrator4/1 -> Sum3/2, r/1, Sum8/2
  Sum8/1 -> Gain4/1
  rudder angle/1 -> Sum1/2
  compass/1 -> Sum2/1
  Sum1/1 -> Gain5/1
  Integrator1/1 -> psi_w/1, Sum4/1, Gain1/1, Sum5/2  "psi_w"
  Sum5/1 -> Integrator2/1  "psi_WF"
  Integrator2/1 -> Gain2/1  "xi_w"
  Gain2/1 -> Sum6/2
  Gain1/1 -> Sum6/3
  Sum6/1 -> Integrator1/1
  Sum4/1 -> Sum2/2
  "[-inf inf] to [-pi pi]1"/1 -> psi/1, Sum4/2
  Integrator/1 -> "[-inf inf] to [-pi pi]1"/1  "psi"
  Sum2/1 -> "[-inf inf] to [-pi pi]"/1
  Sum3/1 -> Integrator/1
  H'/1 -> "  "/1, H'*H/1, P*H'/2  "H'"
  H'*H/1 -> "    "/1
  P*H'/1 -> "     "/1
  "    "/1 -> P*H'*(1/r)*H*P/2
  "  "/1 -> H'*H/2  "H"
  matrices/1(A) -> AP/1

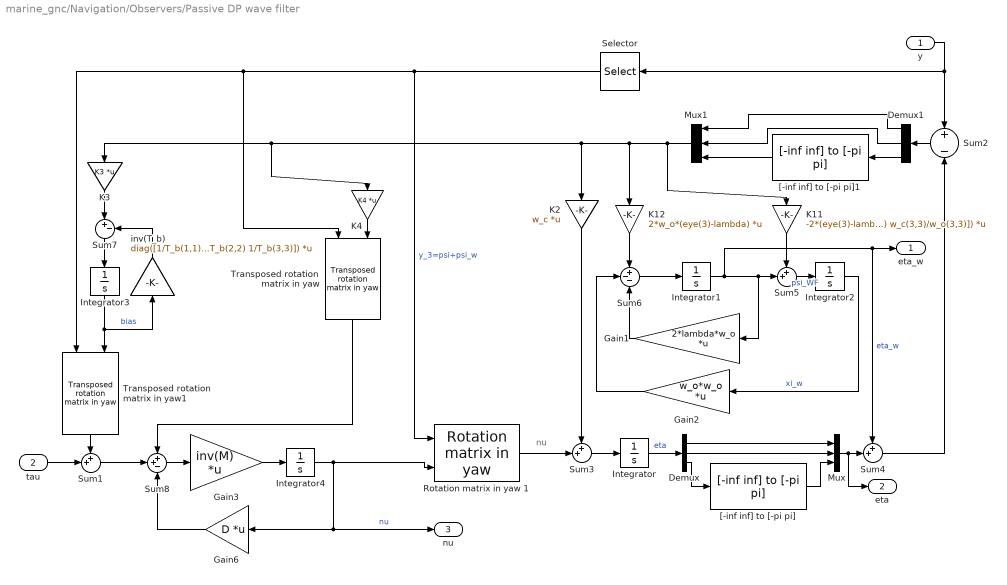
== system marine_gnc/Navigation/Observers/Passive DP wave filter ==
  note: nu
  y : Inport  OutDataType=sfix(16)  OutScaling=2^0
  tau : Inport  Port=2  OutDataType=sfix(16)  OutScaling=2^0
  Demux : Demux  Outputs=3
  Demux1 : Demux  Outputs=3
  Gain1 : Gain  Gain=2*lambda*w_o  Multiplication=Matrix(K*u)  ParameterDataType=sfix(16)  ParameterScaling=2^0  OutDataType=sfix(16)  OutScaling=2^0  SaturateOnIntegerOverflow=on  OutDataTypeStr=Inherit: Same as input  ParamDataTypeStr=Inherit: Same as input
  Gain2 : Gain  Gain=w_o*w_o  Multiplication=Matrix(K*u)  ParameterDataType=sfix(16)  ParameterScaling=2^0  OutDataType=sfix(16)  OutScaling=2^0  SaturateOnIntegerOverflow=on  OutDataTypeStr=Inherit: Same as input  ParamDataTypeStr=Inherit: Same as input
  Gain3 : Gain  Gain=inv(M)  Multiplication=Matrix(K*u)  ParameterDataType=sfix(16)  ParameterScaling=2^0  OutDataType=sfix(16)  OutScaling=2^0  SaturateOnIntegerOverflow=on  OutDataTypeStr=Inherit: Same as input  ParamDataTypeStr=Inherit: Same as input
  Gain6 : Gain  Gain=D  Multiplication=Matrix(K*u)  ParameterDataType=sfix(16)  ParameterScaling=2^0  OutDataType=sfix(16)  OutScaling=2^0  SaturateOnIntegerOverflow=on  OutDataTypeStr=Inherit: Same as input  ParamDataTypeStr=Inherit: Same as input
  Integrator{,1..4} (5 alike) : Integrator
  K11 : Gain  Gain=-2*(eye(3)-lambda)*diag([w_c(1,1)/w_o(1,1) w_c(2,2)/w_o(2,2) w_c(3,3)/w_o(3,3)])  Multiplication=Matrix(K*u)  ParameterDataType=sfix(16)  ParameterScaling=2^0  OutDataType=sfix(16)  OutScaling=2^0  SaturateOnIntegerOverflow=on  OutDataTypeStr=Inherit: Same as input  ParamDataTypeStr=Inherit: Same as input
  K12 : Gain  Gain=2*w_o*(eye(3)-lambda)  Multiplication=Matrix(K*u)  ParameterDataType=sfix(16)  ParameterScaling=2^0  OutDataType=sfix(16)  OutScaling=2^0  SaturateOnIntegerOverflow=on  OutDataTypeStr=Inherit: Same as input  ParamDataTypeStr=Inherit: Same as input
  K2 : Gain  Gain=w_c  Multiplication=Matrix(K*u)  ParameterDataType=sfix(16)  ParameterScaling=2^0  OutDataType=sfix(16)  OutScaling=2^0  SaturateOnIntegerOverflow=on  OutDataTypeStr=Inherit: Same as input  ParamDataTypeStr=Inherit: Same as input
  K3 : Gain  Gain=K3  Multiplication=Matrix(K*u)  ParameterDataType=sfix(16)  ParameterScaling=2^0  OutDataType=sfix(16)  OutScaling=2^0  SaturateOnIntegerOverflow=on  OutDataTypeStr=Inherit: Same as input  ParamDataTypeStr=Inherit: Same as input
  K4 : Gain  Gain=K4  Multiplication=Matrix(K*u)  ParameterDataType=sfix(16)  ParameterScaling=2^0  OutDataType=sfix(16)  OutScaling=2^0  SaturateOnIntegerOverflow=on  OutDataTypeStr=Inherit: Same as input  ParamDataTypeStr=Inherit: Same as input
  Mux : Mux  Inputs=3
  Mux1 : Mux  Inputs=3
  Rotation matrix in yaw 1 : marine_gnc/Models/ Kinematics/Rotation matrix in yaw 
  Selector : Selector  InputPortWidth=3  IndexOptions=Index vector (dialog)  Indices=[3]  OutputSizes=1
  Sum{1,3..5} (4 alike) : Sum  Inputs=++|  OutDataType=sfix(16)  OutScaling=2^0  SaturateOnIntegerOverflow=on  InputSameDT=on  OutDataTypeStr=Inherit: Same as first input
  Sum2 : Sum  Inputs=+|-  OutDataType=sfix(16)  OutScaling=2^0  SaturateOnIntegerOverflow=on  InputSameDT=on  OutDataTypeStr=Inherit: Same as first input
  Sum6 : Sum  Inputs=+--  OutDataType=sfix(16)  OutScaling=2^0  SaturateOnIntegerOverflow=on  InputSameDT=on  OutDataTypeStr=Inherit: Same as first input
  Sum7 : Sum  Inputs=|+-  OutDataType=sfix(16)  OutScaling=2^0  SaturateOnIntegerOverflow=on  InputSameDT=on  OutDataTypeStr=Inherit: Same as first input
  Sum8 : Sum  Inputs=++-  OutDataType=sfix(16)  OutScaling=2^0  SaturateOnIntegerOverflow=on  InputSameDT=on  OutDataTypeStr=Inherit: Same as first input
  Transposed rotation  matrix in yaw : marine_gnc/Models/ Kinematics/Transposed rotation  matrix in yaw
  Transposed rotation  matrix in yaw1 : marine_gnc/Models/ Kinematics/Transposed rotation  matrix in yaw
  "[-inf inf] to [-pi pi]" : marine_gnc/Utilities/Math Operations/[-inf inf] to [-pi pi]
  "[-inf inf] to [-pi pi]1" : marine_gnc/Utilities/Math Operations/[-inf inf] to [-pi pi]
  inv(T_b) : Gain  Gain=diag([1/T_b(1,1) 1/T_b(2,2) 1/T_b(3,3)])  Multiplication=Matrix(K*u)  ParameterDataType=sfix(16)  ParameterScaling=2^0  OutDataType=sfix(16)  OutScaling=2^0  SaturateOnIntegerOverflow=on  OutDataTypeStr=Inherit: Same as input  ParamDataTypeStr=Inherit: Same as input
  eta_w : Outport  OutDataType=sfix(16)  OutScaling=2^0
  eta : Outport  Port=2  OutDataType=sfix(16)  OutScaling=2^0
  nu : Outport  Port=3  OutDataType=sfix(16)  OutScaling=2^0
  wires:
  Sum3/1 -> Integrator/1
  Mux1/1 -> K11/1, K12/1, K2/1, K3/1, K4/1
  Sum4/1 -> Sum2/2
  K2/1 -> Sum3/1
  Sum6/1 -> Integrator1/1
  Gain1/1 -> Sum6/3
  Gain2/1 -> Sum6/2
  Integrator2/1 -> Gain2/1  "xi_w"
  K11/1 -> Sum5/1
  K12/1 -> Sum6/1
  Sum5/1 -> Integrator2/1  "psi_WF"
  Integrator1/1 -> Sum5/2, Gain1/1, Sum4/1, eta_w/1  "eta_w"
  y/1 -> Sum2/1, Selector/1
  tau/1 -> Sum1/2
  Sum7/1 -> Integrator3/1
  Integrator3/1 -> inv(T_b)/1, Transposed rotation  matrix in yaw1/2  "bias"
  inv(T_b)/1 -> Sum7/2
  Integrator/1 -> Demux/1  "eta"
  "[-inf inf] to [-pi pi]"/1 -> Mux/3
  Mux/1 -> Sum4/2, eta/1
  Demux/1 -> Mux/1
  Demux/2 -> Mux/2
  "[-inf inf] to [-pi pi]1"/1 -> Mux1/3
  Demux1/2 -> Mux1/2
  Demux1/3 -> "[-inf inf] to [-pi pi]1"/1
  Sum2/1 -> Demux1/1
  Demux1/1 -> Mux1/1
  Selector/1 -> Transposed rotation  matrix in yaw/1, Transposed rotation  matrix in yaw1/1, Rotation matrix in yaw 1/1  "y_3=psi+psi_w"
  K4/1 -> Transposed rotation  matrix in yaw/2
  Transposed rotation  matrix in yaw/1 -> Sum8/1
  Transposed rotation  matrix in yaw1/1 -> Sum1/1
  K3/1 -> Sum7/1
  Integrator4/1 -> Gain6/1, nu/1, Rotation matrix in yaw 1/2  "nu"
  Rotation matrix in yaw 1/1 -> Sum3/2
  Gain3/1 -> Integrator4/1
  Sum1/1 -> Sum8/2
  Sum8/1 -> Gain3/1
  Gain6/1 -> Sum8/3
  Demux/3 -> "[-inf inf] to [-pi pi]"/1

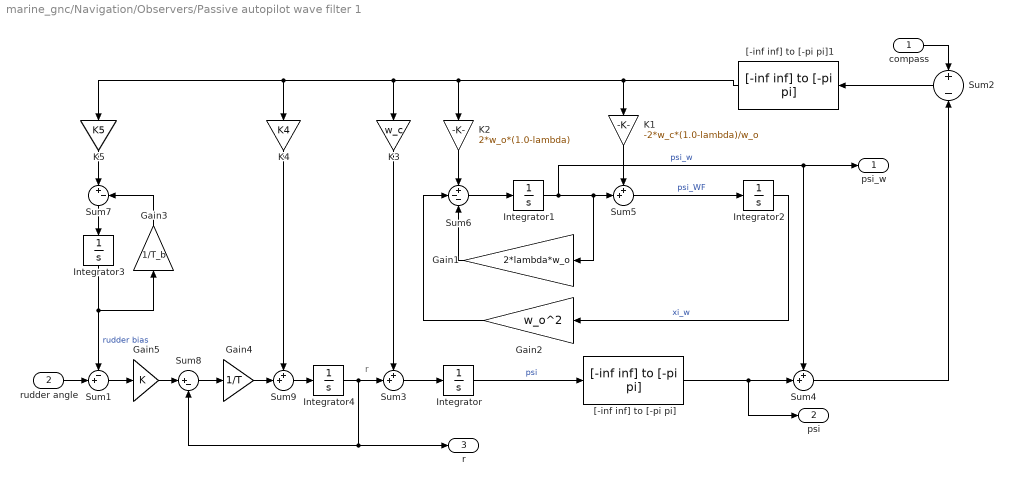
== system marine_gnc/Navigation/Observers/Passive autopilot wave filter 1 ==
  note: r
  compass : Inport  OutDataType=sfix(16)  OutScaling=2^0
  rudder angle : Inport  Port=2  OutDataType=sfix(16)  OutScaling=2^0
  Gain1 : Gain  Gain=2*lambda*w_o  ParameterDataType=sfix(16)  ParameterScaling=2^0  OutDataType=sfix(16)  OutScaling=2^0  SaturateOnIntegerOverflow=on  OutDataTypeStr=Inherit: Same as input  ParamDataTypeStr=Inherit: Same as input
  Gain2 : Gain  Gain=w_o^2  ParameterDataType=sfix(16)  ParameterScaling=2^0  OutDataType=sfix(16)  OutScaling=2^0  SaturateOnIntegerOverflow=on  OutDataTypeStr=Inherit: Same as input  ParamDataTypeStr=Inherit: Same as input
  Gain3 : Gain  Gain=1/T_b  ParameterDataType=sfix(16)  ParameterScaling=2^0  OutDataType=sfix(16)  OutScaling=2^0  SaturateOnIntegerOverflow=on  OutDataTypeStr=Inherit: Same as input  ParamDataTypeStr=Inherit: Same as input
  Gain4 : Gain  Gain=1/T  ParameterDataType=sfix(16)  ParameterScaling=2^0  OutDataType=sfix(16)  OutScaling=2^0  SaturateOnIntegerOverflow=on  OutDataTypeStr=Inherit: Same as input  ParamDataTypeStr=Inherit: Same as input
  Gain5 : Gain  Gain=K  ParameterDataType=sfix(16)  ParameterScaling=2^0  OutDataType=sfix(16)  OutScaling=2^0  SaturateOnIntegerOverflow=on  OutDataTypeStr=Inherit: Same as input  ParamDataTypeStr=Inherit: Same as input
  Integrator{,1..4} (5 alike) : Integrator
  K1 : Gain  Gain=-2*w_c*(1.0-lambda)/w_o  ParameterDataType=sfix(16)  ParameterScaling=2^0  OutDataType=sfix(16)  OutScaling=2^0  SaturateOnIntegerOverflow=on  OutDataTypeStr=Inherit: Same as input  ParamDataTypeStr=Inherit: Same as input
  K2 : Gain  Gain=2*w_o*(1.0-lambda)  ParameterDataType=sfix(16)  ParameterScaling=2^0  OutDataType=sfix(16)  OutScaling=2^0  SaturateOnIntegerOverflow=on  OutDataTypeStr=Inherit: Same as input  ParamDataTypeStr=Inherit: Same as input
  K3 : Gain  Gain=w_c  ParameterDataType=sfix(16)  ParameterScaling=2^0  OutDataType=sfix(16)  OutScaling=2^0  SaturateOnIntegerOverflow=on  OutDataTypeStr=Inherit: Same as input  ParamDataTypeStr=Inherit: Same as input
  K4 : Gain  Gain=K4  ParameterDataType=sfix(16)  ParameterScaling=2^0  OutDataType=sfix(16)  OutScaling=2^0  SaturateOnIntegerOverflow=on  OutDataTypeStr=Inherit: Same as input  ParamDataTypeStr=Inherit: Same as input
  K5 : Gain  Gain=K5  ParameterDataType=sfix(16)  ParameterScaling=2^0  OutDataType=sfix(16)  OutScaling=2^0  SaturateOnIntegerOverflow=on  OutDataTypeStr=Inherit: Same as input  ParamDataTypeStr=Inherit: Same as input
  Sum1 : Sum  Inputs=-+|  OutDataType=sfix(16)  OutScaling=2^0  SaturateOnIntegerOverflow=on  InputSameDT=on  OutDataTypeStr=Inherit: Same as first input
  Sum2 : Sum  Inputs=+|-  OutDataType=sfix(16)  OutScaling=2^0  SaturateOnIntegerOverflow=on  InputSameDT=on  OutDataTypeStr=Inherit: Same as first input
  Sum{3..5,9} (4 alike) : Sum  Inputs=++|  OutDataType=sfix(16)  OutScaling=2^0  SaturateOnIntegerOverflow=on  InputSameDT=on  OutDataTypeStr=Inherit: Same as first input
  Sum6 : Sum  Inputs=+--  OutDataType=sfix(16)  OutScaling=2^0  SaturateOnIntegerOverflow=on  InputSameDT=on  OutDataTypeStr=Inherit: Same as first input
  Sum7 : Sum  Inputs=|+-  OutDataType=sfix(16)  OutScaling=2^0  SaturateOnIntegerOverflow=on  InputSameDT=on  OutDataTypeStr=Inherit: Same as first input
  Sum8 : Sum  Inputs=|+-  OutDataType=sfix(16)  OutScaling=2^0  SaturateOnIntegerOverflow=on  InputSameDT=on  OutDataTypeStr=Inherit: Same as first input
  "[-inf inf] to [-pi pi]" : marine_gnc/Utilities/Math Operations/[-inf inf] to [-pi pi]
  "[-inf inf] to [-pi pi]1" : marine_gnc/Utilities/Math Operations/[-inf inf] to [-pi pi]
  psi_w : Outport  OutDataType=sfix(16)  OutScaling=2^0
  psi : Outport  Port=2  OutDataType=sfix(16)  OutScaling=2^0
  r : Outport  Port=3  OutDataType=sfix(16)  OutScaling=2^0
  wires:
  Sum3/1 -> Integrator/1
  Sum2/1 -> "[-inf inf] to [-pi pi]1"/1
  "[-inf inf] to [-pi pi]1"/1 -> K1/1, K2/1, K3/1, K4/1, K5/1
  Integrator/1 -> "[-inf inf] to [-pi pi]"/1  "psi"
  "[-inf inf] to [-pi pi]"/1 -> Sum4/2, psi/1
  Sum4/1 -> Sum2/2
  K3/1 -> Sum3/1
  Sum6/1 -> Integrator1/1
  Gain1/1 -> Sum6/3
  Gain2/1 -> Sum6/2
  Integrator2/1 -> Gain2/1  "xi_w"
  K1/1 -> Sum5/1
  K2/1 -> Sum6/1
  Sum5/1 -> Integrator2/1  "psi_WF"
  Integrator1/1 -> Sum5/2, Gain1/1, Sum4/1, psi_w/1  "psi_w"
  Sum1/1 -> Gain5/1
  compass/1 -> Sum2/1
  rudder angle/1 -> Sum1/2
  Sum8/1 -> Gain4/1
  Integrator4/1 -> Sum8/2, r/1, Sum3/2
  K5/1 -> Sum7/1
  Sum7/1 -> Integrator3/1
  Integrator3/1 -> Sum1/1, Gain3/1  "rudder bias"
  Gain3/1 -> Sum7/2
  Gain5/1 -> Sum8/1
  Gain4/1 -> Sum9/2
  Sum9/1 -> Integrator4/1
  K4/1 -> Sum9/1

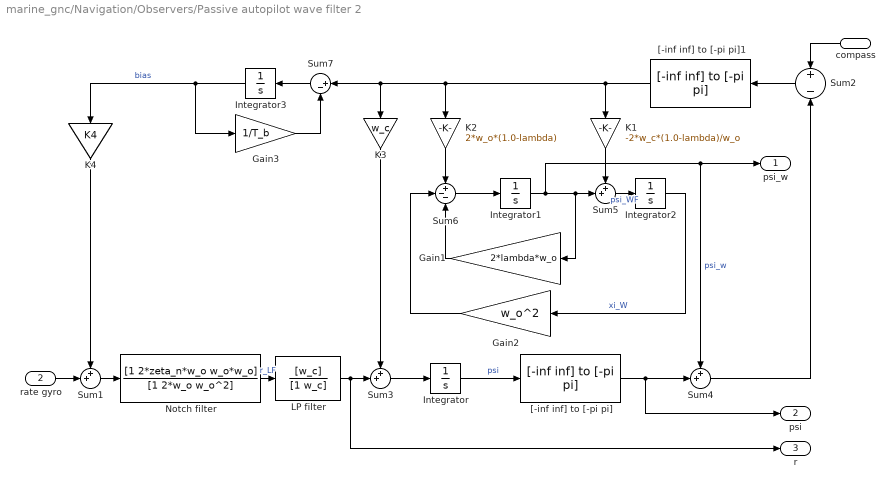
== system marine_gnc/Navigation/Observers/Passive autopilot wave filter 2 ==
  compass : Inport  OutDataType=sfix(16)  OutScaling=2^0
  rate gyro : Inport  Port=2  OutDataType=sfix(16)  OutScaling=2^0
  Gain1 : Gain  Gain=2*lambda*w_o  ParameterDataType=sfix(16)  ParameterScaling=2^0  OutDataType=sfix(16)  OutScaling=2^0  SaturateOnIntegerOverflow=on  OutDataTypeStr=Inherit: Same as input  ParamDataTypeStr=Inherit: Same as input
  Gain2 : Gain  Gain=w_o^2  ParameterDataType=sfix(16)  ParameterScaling=2^0  OutDataType=sfix(16)  OutScaling=2^0  SaturateOnIntegerOverflow=on  OutDataTypeStr=Inherit: Same as input  ParamDataTypeStr=Inherit: Same as input
  Gain3 : Gain  Gain=1/T_b  ParameterDataType=sfix(16)  ParameterScaling=2^0  OutDataType=sfix(16)  OutScaling=2^0  SaturateOnIntegerOverflow=on  OutDataTypeStr=Inherit: Same as input  ParamDataTypeStr=Inherit: Same as input
  Integrator{,1..3} (4 alike) : Integrator
  K1 : Gain  Gain=-2*w_c*(1.0-lambda)/w_o  ParameterDataType=sfix(16)  ParameterScaling=2^0  OutDataType=sfix(16)  OutScaling=2^0  SaturateOnIntegerOverflow=on  OutDataTypeStr=Inherit: Same as input  ParamDataTypeStr=Inherit: Same as input
  K2 : Gain  Gain=2*w_o*(1.0-lambda)  ParameterDataType=sfix(16)  ParameterScaling=2^0  OutDataType=sfix(16)  OutScaling=2^0  SaturateOnIntegerOverflow=on  OutDataTypeStr=Inherit: Same as input  ParamDataTypeStr=Inherit: Same as input
  K3 : Gain  Gain=w_c  ParameterDataType=sfix(16)  ParameterScaling=2^0  OutDataType=sfix(16)  OutScaling=2^0  SaturateOnIntegerOverflow=on  OutDataTypeStr=Inherit: Same as input  ParamDataTypeStr=Inherit: Same as input
  K4 : Gain  Gain=K4  ParameterDataType=sfix(16)  ParameterScaling=2^0  OutDataType=sfix(16)  OutScaling=2^0  SaturateOnIntegerOverflow=on  OutDataTypeStr=Inherit: Same as input  ParamDataTypeStr=Inherit: Same as input
  LP filter : TransferFcn  Numerator=[w_c]  Denominator=[1 w_c]
  Notch filter : TransferFcn  Numerator=[1 2*zeta_n*w_o w_o*w_o]  Denominator=[1 2*w_o w_o^2]
  Sum{1,3..5} (4 alike) : Sum  Inputs=++|  OutDataType=sfix(16)  OutScaling=2^0  SaturateOnIntegerOverflow=on  InputSameDT=on  OutDataTypeStr=Inherit: Same as first input
  Sum2 : Sum  Inputs=+|-  OutDataType=sfix(16)  OutScaling=2^0  SaturateOnIntegerOverflow=on  InputSameDT=on  OutDataTypeStr=Inherit: Same as first input
  Sum6 : Sum  Inputs=+--  OutDataType=sfix(16)  OutScaling=2^0  SaturateOnIntegerOverflow=on  InputSameDT=on  OutDataTypeStr=Inherit: Same as first input
  Sum7 : Sum  Inputs=|+-  OutDataType=sfix(16)  OutScaling=2^0  SaturateOnIntegerOverflow=on  InputSameDT=on  OutDataTypeStr=Inherit: Same as first input
  "[-inf inf] to [-pi pi]" : marine_gnc/Utilities/Math Operations/[-inf inf] to [-pi pi]
  "[-inf inf] to [-pi pi]1" : marine_gnc/Utilities/Math Operations/[-inf inf] to [-pi pi]
  psi_w : Outport  OutDataType=sfix(16)  OutScaling=2^0
  psi : Outport  Port=2  OutDataType=sfix(16)  OutScaling=2^0
  r : Outport  Port=3  OutDataType=sfix(16)  OutScaling=2^0
  wires:
  K4/1 -> Sum1/1
  Sum3/1 -> Integrator/1
  Sum2/1 -> "[-inf inf] to [-pi pi]1"/1
  "[-inf inf] to [-pi pi]1"/1 -> K1/1, K2/1, K3/1, Sum7/1
  Integrator/1 -> "[-inf inf] to [-pi pi]"/1  "psi"
  "[-inf inf] to [-pi pi]"/1 -> Sum4/2, psi/1
  Sum4/1 -> Sum2/2
  K3/1 -> Sum3/1
  Sum6/1 -> Integrator1/1
  Gain1/1 -> Sum6/3
  Gain2/1 -> Sum6/2
  Integrator2/1 -> Gain2/1  "xi_W"
  K1/1 -> Sum5/1
  K2/1 -> Sum6/1
  Sum5/1 -> Integrator2/1  "psi_WF"
  Integrator1/1 -> Sum5/2, Gain1/1, Sum4/1, psi_w/1  "psi_w"
  Integrator3/1 -> Gain3/1, K4/1  "bias"
  Notch filter/1 -> LP filter/1  "r_LF"
  Sum1/1 -> Notch filter/1
  LP filter/1 -> Sum3/2, r/1
  Sum7/1 -> Integrator3/1
  Gain3/1 -> Sum7/2
  compass/1 -> Sum2/1
  rate gyro/1 -> Sum1/2

== system marine_gnc/Utilities/Dynamics/2nd order time constant ==
  In : Inport  OutDataType=sfix(16)  OutScaling=2^0
  Transfer Fcn1 : TransferFcn  Denominator=[1/(1.5/T)^2 2/(1.5/T) 1]
  Out : Outport  OutDataType=sfix(16)  OutScaling=2^0
  wires:
  In/1 -> Transfer Fcn1/1
  Transfer Fcn1/1 -> Out/1

== system marine_gnc/Utilities/Math Operations/Unit Conversion ==
  In : Inport  OutDataType=sfix(16)  OutScaling=2^0
  Gain : Gain  Gain=k  ParameterDataType=sfix(16)  ParameterScaling=2^0  OutDataType=sfix(16)  OutScaling=2^0  SaturateOnIntegerOverflow=on  OutDataTypeStr=Inherit: Same as input  ParamDataTypeStr=Inherit: Same as input
  Out : Outport  OutDataType=sfix(16)  OutScaling=2^0
  wires:
  In/1 -> Gain/1
  Gain/1 -> Out/1
